simulink model "model2_RegulatorDesign"  (R2020a)
settings: Solver=FixedStepAuto  StartTime=0.0  StopTime=T  FixedStep=Ts  RelTol=1e-3
undefined symbols (not defined in the file): K, L, omgn, Ts, x0
settings Model: Creator=XiaoCY  LastModifiedBy=XiaoCY
settings DataIOCC: ReturnWorkspaceOutputs=off

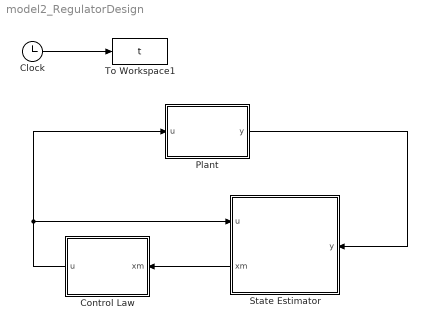
== system model2_RegulatorDesign ==
  Clock : Clock
  Control Law : Subsystem
  Plant : Subsystem
  State Estimator : Subsystem
      settings: PortSchema="{\"entries\":[{\"content\":{\"sides\":[{\"content\":{\"connectorIds\":[\"In1\"]},\"type\":\"ConnectorPlacement.EquallySpacedRectSide\",\"uuid\":\"995efd48-3db5-4a6e-85f6-a349d6a63930\"},{\"content\":{\"connectorIds\":[\"In2\",\"Out1\"],\"side\":\"RIGHT\"},\"type\":\"ConnectorPlacement.EquallySpacedRectSide\",\"uuid\":\"626e22d4-5752-4239-b2ce-472c77ace920\"},{\"content\":{\"connectorIds\":[],\"side\":\"TOP\"},\"type\":\"ConnectorPlacement.EquallySpacedRectSide\",\"uuid\":\"cb599412-420c-4014-940e-49f432b7cbea\"}]},\"type\":\"ConnectorPlacement.EquallySpacedConnector\",\"uuid\":\"e0cccee1-86a0-41f4-a3e5-9044b1b28e69\"}],\"packageUris\":[\"http://schema.mathworks.com/mf0/Connector/19700101\"],\"version\":\"1.0\"}"
  To Workspace1 : ToWorkspace  VariableName=t  SampleTime=Ts
  wires:
  Clock/1 -> To Workspace1/1
  Plant/1(y) -> State Estimator/1(y)
  State Estimator/1(xm) -> Control Law/1(xm)
  Control Law/1(u) -> Plant/1(u), State Estimator/2(u)

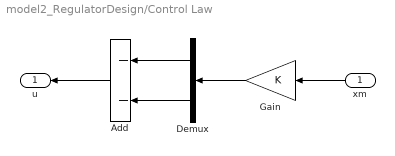
== system model2_RegulatorDesign/Control Law ==
  xm : Inport
  Add : Sum  Inputs=--
  Demux : Demux  Outputs=2
  Gain : Gain  Gain=K
  u : Outport
  wires:
  xm/1 -> Gain/1
  Demux/2 -> Add/2
  Add/1 -> u/1
  Gain/1 -> Demux/1
  Demux/1 -> Add/1

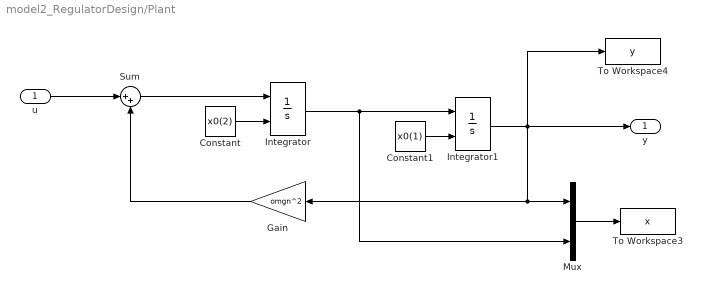
== system model2_RegulatorDesign/Plant ==
  u : Inport
  Constant : Constant  Value=x0(2)
  Constant1 : Constant  Value=x0(1)
  Gain : Gain  Gain=omgn^2
  Integrator : Integrator  InitialConditionSource=external
  Integrator1 : Integrator  InitialConditionSource=external
  Mux : Mux  Inputs=2
  Sum : Sum  Inputs=|++
  To Workspace3 : ToWorkspace  VariableName=x  SampleTime=Ts
  To Workspace4 : ToWorkspace  VariableName=y  SampleTime=Ts
  y : Outport
  wires:
  Integrator/1 -> Mux/2, Integrator1/1
  Constant1/1 -> Integrator1/2
  u/1 -> Sum/1
  Constant/1 -> Integrator/2
  Sum/1 -> Integrator/1
  Gain/1 -> Sum/2
  Mux/1 -> To Workspace3/1
  Integrator1/1 -> Gain/1, Mux/1, To Workspace4/1, y/1

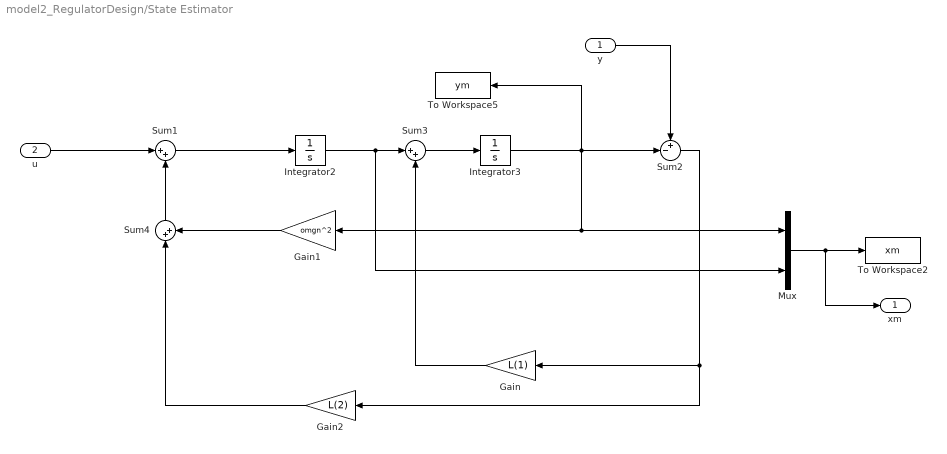
== system model2_RegulatorDesign/State Estimator ==
  y : Inport
  u : Inport  Port=2
  Gain : Gain  Gain=L(1)
  Gain1 : Gain  Gain=omgn^2
  Gain2 : Gain  Gain=L(2)
  Integrator2 : Integrator
  Integrator3 : Integrator
  Mux : Mux  Inputs=2
  Sum1 : Sum  Inputs=|++
  Sum2 : Sum  Inputs=+-|
  Sum3 : Sum  Inputs=|++
  Sum4 : Sum  Inputs=|++
  To Workspace2 : ToWorkspace  VariableName=xm  SampleTime=Ts
  To Workspace5 : ToWorkspace  VariableName=ym  SampleTime=Ts
  xm : Outport
  wires:
  y/1 -> Sum2/1
  Integrator3/1 -> Sum2/2, To Workspace5/1, Mux/1, Gain1/1
  Sum1/1 -> Integrator2/1
  u/1 -> Sum1/1
  Integrator2/1 -> Mux/2, Sum3/1
  Mux/1 -> xm/1, To Workspace2/1
  Sum2/1 -> Gain2/1, Gain/1
  Sum3/1 -> Integrator3/1
  Gain1/1 -> Sum4/2
  Sum4/1 -> Sum1/2
  Gain/1 -> Sum3/2
  Gain2/1 -> Sum4/1
